simulink model "MRAC_Ideal"  (R2021b)
settings: Solver=VariableStepAuto  StartTime=0.0  StopTime=TF  RelTol=1e-3
values from neighbouring files (symbols this model uses):
  Amplitude = 1/pi    (= 0.318309886184)    [Runner.m]
  Frequency = 1    [Runner.m]
  Phi = tanh(360/pi * q)    [AdaptiveLaws.m]    (also in Dynamics.m; Phi.m; u_ideal.m)
  q0 = .001    (= 0.001)    [Runner.m]
  u_ideal = (1/Md) * ( ((a_ref - Mq) * q) + (b_ref * q_cmd)) - f    [u_ideal.m]
undefined symbols (not defined in the file or in its folder): Dynamics
settings Model: Creator=maklenestrada  LastModifiedBy=maklenestrada

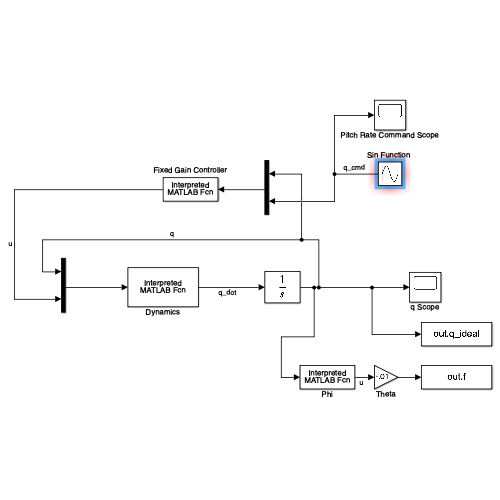
[thumbnail: Simulink's stored preview of the top-level diagram]
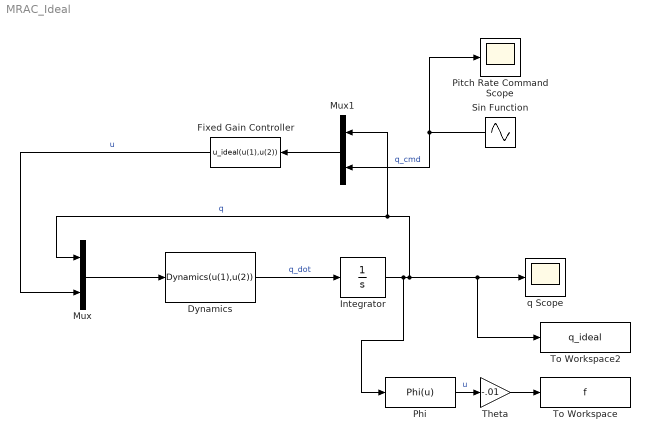
== system MRAC_Ideal ==
  Dynamics : MATLABFcn  MATLABFcn=Dynamics(u(1),u(2))
  Fixed Gain Controller : MATLABFcn  MATLABFcn=u_ideal(u(1),u(2))
  Integrator : Integrator  InitialCondition=q0
  Mux : Mux  Inputs=2
  Mux1 : Mux  Inputs=2
  Phi : MATLABFcn  MATLABFcn=Phi(u)
  Pitch Rate Command Scope : Scope
  "Sin Function " : Sin  Amplitude=Amplitude  Frequency=Frequency  SampleTime=0
  Theta : Gain  Gain=-.01
  To Workspace : ToWorkspace  VariableName=f  SaveFormat=Timeseries  SampleTime=-1
  To Workspace2 : ToWorkspace  VariableName=q_ideal  SaveFormat=Timeseries  SampleTime=-1
  q Scope : Scope
  wires:
  "Sin Function "/1 -> Mux1/2, Pitch Rate Command Scope/1  "q_cmd"
  Integrator/1 -> To Workspace2/1, q Scope/1, Mux1/1, Mux/1, Phi/1  "q"
  Dynamics/1 -> Integrator/1  "q_dot"
  Mux/1 -> Dynamics/1
  Fixed Gain Controller/1 -> Mux/2  "u"
  Mux1/1 -> Fixed Gain Controller/1
  Phi/1 -> Theta/1  "u"
  Theta/1 -> To Workspace/1
